simulink model "BrainBF"  (R2019a)
settings: Solver=VariableStepAuto  StartTime=0.0  StopTime=10.0  RelTol=1e-3
undefined symbols (not defined in the file): GBT_B, r_BGU, T_gB, V_gBF
settings Model: Creator=jcp2  LastModifiedBy=rache

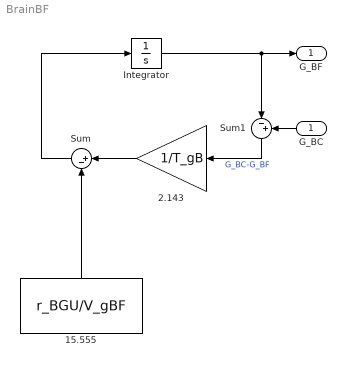
== system BrainBF ==
  G_BC : Inport
  15.555 : Constant  Value=r_BGU/V_gBF
  2.143 : Gain  Gain=1/T_gB
  Integrator : Integrator  InitialCondition=GBT_B  LimitOutput=on  LowerSaturationLimit=0
  Sum : Sum  Inputs=|+-
  Sum1 : Sum  Inputs=|-+
  G_BF : Outport
  wires:
  Integrator/1 -> Sum1/1, G_BF/1
  G_BC/1 -> Sum1/2
  Sum1/1 -> 2.143/1  "G_BC-G_BF"
  2.143/1 -> Sum/1
  15.555/1 -> Sum/2
  Sum/1 -> Integrator/1
